simulink model "e1_1"  (R2022a)
settings: Solver=VariableStepAuto  StartTime=0.0  StopTime=25  RelTol=1e-3
undefined symbols (not defined in the file or in its folder): sigbuilder_block
libraries: simulink_extras x4
settings Model: Creator=18075  LastModifiedBy=18075

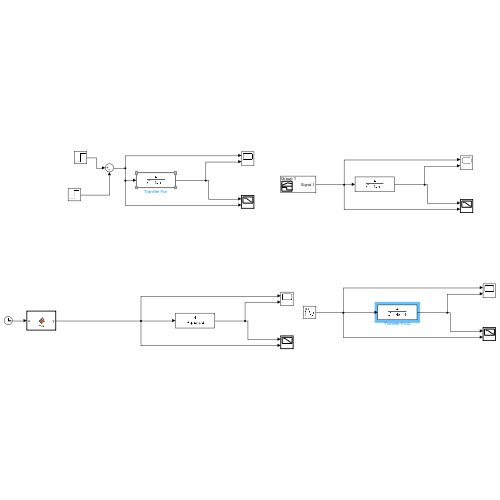
[thumbnail: Simulink's stored preview of the top-level diagram]
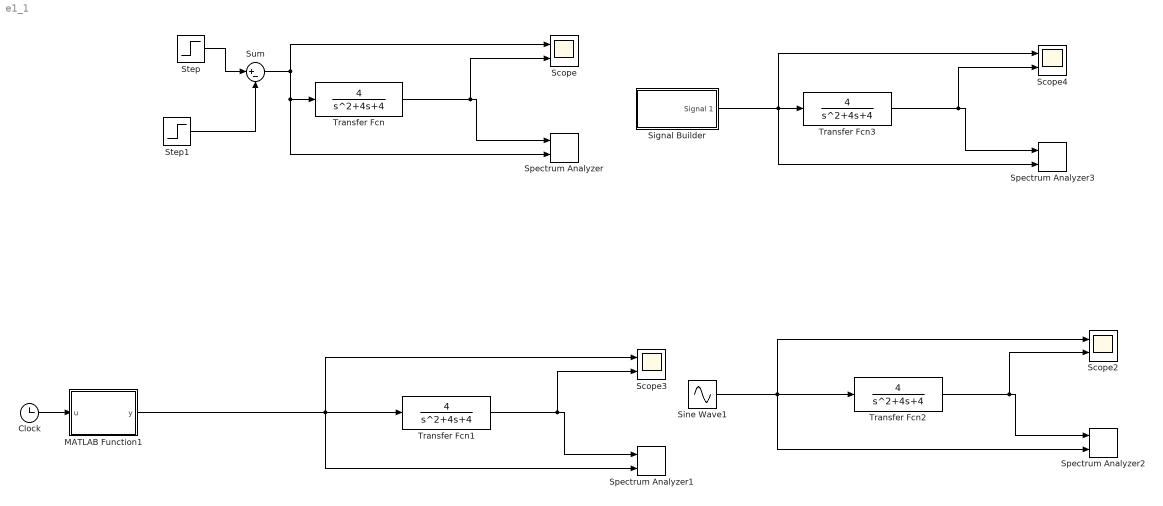
== system e1_1 ==
  Clock : Clock
  MATLAB Function1 : MATLAB Function  TreatAsAtomicUnit=on
  Scope{,2..4} (4 alike) : Scope  NumInputPorts=2
  Signal Builder : Subsystem  Tag=STV Subsys  LoadFcn=sigbuilder_block('load');  StartFcn=sigbuilder_block('start');  StopFcn=sigbuilder_block('stop');  ClipboardFcn=sigbuilder_block('clipboard');  mask(Sigbuilder block){tuvar=[0:10]}
      mask help: Simulink:masks:SigbuilderBlock_MD
      mask init:
      | if ~strcmp(get_param(bdroot(gcbh),'SimulationStatus'),'stopped') tuvar = sigbuilder_block('maskInit'); end
      settings: CopyFcn=sigbuilder_block('copy');  DeleteFcn=sigbuilder_block('delete');  ModelCloseFcn=sigbuilder_block('modelClose');  PreSaveFcn=sigbuilder_block('preSave');  PauseFcn=sigbuilder_block('pause');  ContinueFcn=sigbuilder_block('continue');  NameChangeFcn=sigbuilder_block('namechange');  OpenFcn=sigbuilder_block('open',[437.6 199.2 550.4 400 ]);  CloseFcn=sigbuilder_block('close');
      mask Display: plot(0, 0, 100, 100,[2, 2, 32, 32, 2], [68, 8, 8, 68, 68],[32, 2], [38, 38], [32, 19, 2],[53, 60, 44], [32, 17, 17, 2],[16, 16, 31, 31]);txt = getActiveGroup(gcbh);text(2, 100, txt,'verticalAlignment', 'top');
  Sine Wave1 : Sin  SampleTime=0
  Spectrum Analyzer : simulink_extras/Additional Sinks/Spectrum Analyzer  npts=4096  fftpts=4096  HowOften=512  sampleT=0.01
      settings: SourceProductBaseCode=SL
  Spectrum Analyzer1 : simulink_extras/Additional Sinks/Spectrum Analyzer  npts=4096  fftpts=4096  HowOften=64  sampleT=0.01
      settings: SourceProductBaseCode=SL
  Spectrum Analyzer2 : simulink_extras/Additional Sinks/Spectrum Analyzer  npts=4096  fftpts=4096  HowOften=64  sampleT=0.01
      settings: SourceProductBaseCode=SL
  Spectrum Analyzer3 : simulink_extras/Additional Sinks/Spectrum Analyzer  npts=4096  fftpts=4096  HowOften=512  sampleT=0.01
      settings: SourceProductBaseCode=SL
  Step : Step  SampleTime=0
  Step1 : Step  Time=2  SampleTime=0
  Sum : Sum  Inputs=|+-
  Transfer Fcn{,1..3} (4 alike) : TransferFcn  Numerator=[4]  Denominator=[1 4 4]
  wires:
  Transfer Fcn/1 -> Scope/2, Spectrum Analyzer/1
  Step/1 -> Sum/1
  Sum/1 -> Spectrum Analyzer/2, Transfer Fcn/1, Scope/1
  Step1/1 -> Sum/2
  Transfer Fcn1/1 -> Scope3/2, Spectrum Analyzer1/1
  MATLAB Function1/1(y) -> Scope3/1, Spectrum Analyzer1/2, Transfer Fcn1/1
  Transfer Fcn2/1 -> Scope2/2, Spectrum Analyzer2/1
  Sine Wave1/1 -> Scope2/1, Spectrum Analyzer2/2, Transfer Fcn2/1
  Transfer Fcn3/1 -> Scope4/2, Spectrum Analyzer3/1
  Signal Builder/1(Signal 1) -> Scope4/1, Spectrum Analyzer3/2, Transfer Fcn3/1
  Clock/1 -> MATLAB Function1/1(u)

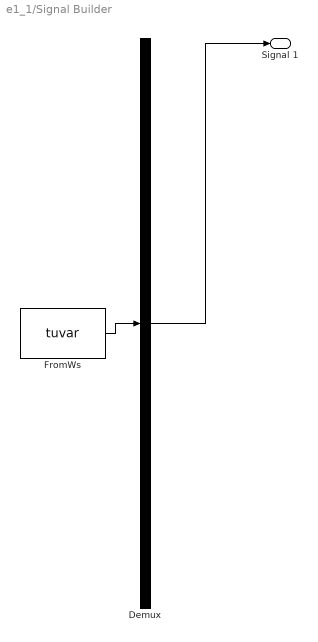
== system e1_1/Signal Builder ==
  Demux : Demux  Tag=STV Demux  Outputs=1
      settings: DisplayOption=none
  FromWs : FromWorkspace  Tag=STV FromWs  VariableName=tuvar
      SigBuilderData=|
      | common.afterFinalStr = 'Extrapolate'
      | common.sampleTime = 0
      | dataSet.timeRange = [0 10]
      | dataSet.name = 'Group 1'
      | sbobj.Groups.Name = 'Group 1'
      | sbobj.Groups.Signals.Name = 'Signal 1'
      | sbobj.Groups.Signals.XData = [0 1 1 4 10]
      | sbobj.Groups.Signals.YData = [0 0 1 0 0]
  Signal 1 : Outport  Tag=STV Outport
  wires:
  Demux/1 -> Signal 1/1
  FromWs/1 -> Demux/1

== matlab function e1_1/MATLAB Function1 ==
  data: u input; y output
function y = fcn(u)
%#codegen

y = exp(-u);
